simulink model "integracionExperimental"  (R2023b)
settings: Solver=VariableStepAuto  StartTime=0.0  StopTime=10.0  RelTol=1e-3
settings Model: Creator=Hajar  LastModifiedBy=Hajar

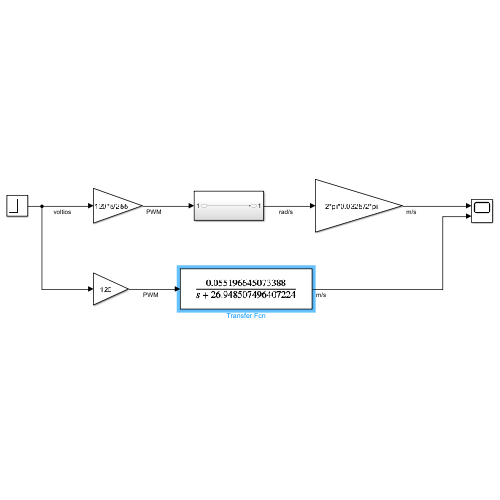
[thumbnail: Simulink's stored preview of the top-level diagram]
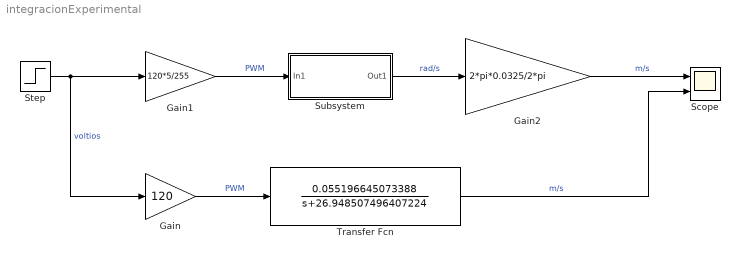
== system integracionExperimental ==
  Gain : Gain  Gain=120
  Gain1 : Gain  Gain=120*5/255
  Gain2 : Gain  Gain=2*pi*0.0325/2*pi
  Scope : Scope  NumInputPorts=2
  Step : Step  SampleTime=0
  Subsystem : Subsystem
  Transfer Fcn : TransferFcn  Numerator=0.055196645073388  Denominator=[1,26.948507496407224]
  wires:
  Gain2/1 -> Scope/1  "m/s"
  Transfer Fcn/1 -> Scope/2  "m/s"
  Gain1/1 -> Subsystem/1(In1)  "PWM"
  Step/1 -> Gain/1, Gain1/1  "voltios"
  Subsystem/1(Out1) -> Gain2/1  "rad/s"
  Gain/1 -> Transfer Fcn/1  "PWM"

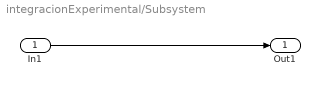
== system integracionExperimental/Subsystem ==
  In1 : Inport
  Out1 : Outport
  wires:
  In1/1 -> Out1/1
